simulink model "RefModel_Control"  (R2019b)
settings: Solver=ode1  StartTime=0.0  StopTime=10.0  FixedStep=dt  RelTol=1e-3
(part 2 of 2)

== matlab function RefModel_Control/input_euler_angle_roll_pitch_euler_rate_yaw4 ==
  data: gains_I_pitch data_store_memory; gains_tau_pitch data_store_memory; gains_P_pitch data_store_memory; gains_D_pitch data_store_memory; gains_imax_pitch data_store_memory; gains_FF_pitch data_store_memory; airspeed_min data_store_memory; last_out_pitch data_store_memory; pid_info_I_pitch data_store_memory; pid_info_P_pitch data_store_memory; pid_info_FF_pitch data_store_memory; pid_info_D_pitch data_store_memory; pid_info_desired_pitch data_store_memory; pid_info_actual_pitch data_store_memory; roll data_store_memory; pitch data_store_memory; roll_limit_cd data_store_memory; aspeed data_store_memory; max_rate_neg data_store_memory; gains_rmax_pitch data_store_memory; GRAVITY_MSS data_store_memory; roll_ff_pitch data_store_memory; HD data_store_memory; gains_D_roll data_store_memory; gains_FF_roll data_store_memory; gains_I_roll data_store_memory; gains_imax_roll data_store_memory; gains_P_roll data_store_memory; gains_rmax_roll data_store_memory; gains_tau_roll data_store_memory; last_out_roll data_store_memory; pid_info_actual_roll data_store_memory; pid_info_D_roll data_store_memory; pid_info_desired_roll data_store_memory; pid_info_FF_roll data_store_memory; pid_info_I_roll data_store_memory; pid_info_P_roll data_store_memory; accel_y data_store_memory; imax_yaw data_store_memory; integrator_yaw data_store_memory; K_A_yaw data_store_memory; K_D_last_yaw data_store_memory; K_D_yaw data_store_memory; K_FF_yaw data_store_memory; K_I_yaw data_store_memory; last_out_yaw data_store_memory; last_rate_hp_in_yaw data_store_memory; last_rate_hp_out_yaw data_store_memory; pid_info_D_yaw data_store_memory; pid_info_I_yaw data_store_memory; throttle_dem data_store_memory; pitch_dem data_store_memory; pitch_limit_min_cd data_store_memory; pitch_limit_max_cd data_store_memory; nav_pitch_cd data_store_memory; inverted_flight data_store_memory; k_rudder data_store_memory; k_aileron data_store_memory; k_throttle data_store_memory; k_elevator data_store_memory; kff_throttle_to_pitch data_store_memory; highest_airspeed data_store_memory; scaling_speed data_store_memory; airspeed_max data_store_memory; latAccDem data_store_memory; smoothed_airspeed data_store_memory; aerodynamic_load_factor data_store_memory; kff_rudder_mix data_store_memory; TASmax data_store_memory; SKE_dem data_store_memory; TASmin data_store_memory; SPE_dem data_store_memory; SPE_est data_store_memory; SKE_est data_store_memory; STE_error data_store_memory; SPEdot_dem data_store_memory; SKEdot_dem data_store_memory; STEdot_min data_store_memory; STEdot_max data_store_memory; SPEdot data_store_memory; SKEdot data_store_memory; STEdotErrLast data_store_memory; timeConstant data_store_memory; throttle_cruise data_store_memory; rot_body_to_ned data_store_memory; rollComp data_store_memory; THRmaxf data_store_memory; THRminf data_store_memory; thrDamp data_store_memory; throttle_slewrate data_store_memory; last_throttle_dem data_store_memory; integGain data_store_memory; integTHR_state data_store_memory; maxClimbRate data_store_memory; minSinkRate data_store_memory; EAS_dem data_store_memory; hgt_dem data_store_memory; throttle_max data_store_memory; throttle_min data_store_memory; pitch_max data_store_memory; PITCHmaxf data_store_memory; pitch_min data_store_memory; PITCHminf data_store_memory; pitch_max_limit data_store_memory; TAS_dem data_store_memory; EAS2TAS data_store_memory; TAS_state data_store_memory; integDTAS_state data_store_memory; spdCompFiltOmega data_store_memory; vel_dot data_store_memory; TAS_dem_adj data_store_memory; TAS_rate_dem data_store_memory; hgt_dem_in_old data_store_memory; maxSinkRate data_store_memory; hgt_dem_prev data_store_memory; hgt_dem_adj_last data_store_memory; hgt_dem_adj data_store_memory; hgt_rate_dem data_store_memory; height data_store_memory; climb_rate data_store_memory; spdWeight data_store_memory; ptchDamp data_store_memory; pitch_dem_unc data_store_memory; integSEB_state data_store_memory; vertAccLim data_store_memory; last_pitch_dem data_store_memory; L1_damping data_store_memory; L1_period data_store_memory; current_loc data_store_memory; groundspeed_vector data_store_memory; target_bearing_cd data_store_memory; L1_dist data_store_memory; crosstrack_error data_store_memory; nav_bearing data_store_memory; L1_xtrack_i_gain data_store_memory; L1_xtrack_i_gain_prev data_store_memory; L1_xtrack_i data_store_memory; last_Nu data_store_memory; WPcircle data_store_memory; data_is_stale data_store_memory; bearing_error data_store_memory; LOCATION_SCALING_FACTOR data_store_memory; yaw data_store_memory; reverse data_store_memory; loiter_bank_limit data_store_memory; dt data_store_memory; roll_limit_cd_inint data_store_memory; accel_x data_store_memory; accel_z data_store_memory; Vz data_store_memory; vdot_filter data_store_memory; pwm_min data_store_memory; pwm_max data_store_memory; pwm_out data_store_memory; LOCATION_SCALING_FACTOR_INV data_store_memory; recalc_leash_z data_store_memory; leash_up_z data_store_memory; POSCONTROL_SPEED_UP data_store_memory; POSCONTROL_ACCEL_Z data_store_memory; POSCONTROL_POS_Z_P data_store_memory; leash_down_z data_store_memory; POSCONTROL_SPEED_DOWN data_store_memory; POSCONTROL_ACCELERATION_MIN data_store_memory; POSCONTROL_LEASH_LENGTH_MIN data_store_memory; limit_pos_up data_store_memory; limit_pos_down data_store_memory; pos_error data_store_memory; pos_target data_store_memory; curr_alt data_store_memory; vel_target data_store_memory; limit_vel_up data_store_memory; limit_vel_down data_store_memory; use_desvel_ff_z data_store_memory; reset_rate_to_accel_z data_store_memory; vel_desired data_store_memory; accel_desired data_store_memory; POSCONTROL_VEL_ERROR_CUTOFF_FREQ data_store_memory; vel_last data_store_memory; freeze_ff_z data_store_memory; vel_error data_store_memory; vel_error_input data_store_memory; curr_vel data_store_memory; accel_target data_store_memory; POSCONTROL_VEL_Z_P data_store_memory; reset_accel_to_throttle data_store_memory; accel_error data_store_memory; z_accel_meas data_store_memory; pid_accel_z_reset_filter data_store_memory; POSCONTROL_ACC_Z_FILT_HZ data_store_memory; pid_accel_z_input data_store_memory; pid_accel_z_derivative data_store_memory; POSCONTROL_ACC_Z_P data_store_memory; pid_accel_z_integrator data_store_memory; POSCONTROL_ACC_Z_IMAX data_store_memory; throttle_hover data_store_memory; throttle_lower data_store_memory; throttle_upper data_store_memory; POSCONTROL_ACC_Z_D data_store_memory; POSCONTROL_ACC_Z_I data_store_memory; throttle_thrust_max data_store_memory; althold_lean_angle_max data_store_memory; angle_limit_tc data_store_memory; angle_boost_enabled data_store_memory; angle_boost data_store_memory; throttle_rpy_mix data_store_memory; throttle_avg_max data_store_memory; AC_ATTITUDE_CONTROL_ANGLE_LIMIT_THROTTLE_MAX data_store_memory; POSCONTROL_POS_XY_P data_store_memory; curr_pos data_store_memory; leash data_store_memory; POSCONTROL_ACCEL_XY data_store_memory; POSCONTROL_VEL_XY_FILT_HZ data_store_memory; POSCONTROL_VEL_XY_FILT_D_HZ data_store_memory; pid_vel_xy_reset_filter data_store_memory; pid_vel_xy_input data_store_memory; pid_vel_xy_derivative data_store_memory; pid_vel_xy_integrator data_store_memory; POSCONTROL_VEL_XY_P data_store_memory; limit_accel_xy data_store_memory; motors_limit_throttle_upper data_store_memory; POSCONTROL_VEL_XY_I data_store_memory; POSCONTROL_VEL_XY_IMAX data_store_memory; POSCONTROL_VEL_XY_D data_store_memory; reset_accel_to_lean_xy data_store_memory; POSCONTROL_ACCEL_FILTER_HZ data_store_memory; accel_xy_input data_store_memory; accel_xy_angle_max data_store_memory; roll_target data_store_memory; pitch_target data_store_memory; POSCONTROL_ACCEL_XY_MAX data_store_memory; recalc_leash_xy data_store_memory; POSCONTROL_SPEED data_store_memory; reset_desired_vel_to_pos data_store_memory; POSCONTROL_OVERSPEED_GAIN_Z data_store_memory; POSCONTROL_JERK_RATIO data_store_memory; accel_last_z_cms data_store_memory; is_active_z data_store_memory; POSCONTROL_STOPPING_DIST_DOWN_MAX data_store_memory; POSCONTROL_STOPPING_DIST_UP_MAX data_store_memory; is_active_xy data_store_memory; attitude_target_quat data_store_memory; attitude_target_ang_vel data_store_memory; thrust_error_angle data_store_memory; rate_target_ang_vel data_store_memory; gyro_z data_store_memory; ang_vel_roll_max data_store_memory; ang_vel_pitch_max data_store_memory; ang_vel_yaw_max data_store_memory; AC_ATTITUDE_THRUST_ERROR_ANGLE data_store_memory; rate_bf_ff_enabled data_store_memory; attitude_ang_error data_store_memory; p_angle_yaw data_store_memory; AC_ATTITUDE_ACCEL_Y_CONTROLLER_MAX_RADSS data_store_memory; use_sqrt_controller data_store_memory; p_angle_roll data_store_memory; AC_ATTITUDE_ACCEL_RP_CONTROLLER_MIN_RADSS data_store_memory; AC_ATTITUDE_ACCEL_RP_CONTROLLER_MAX_RADSS data_store_memory; p_angle_pitch data_store_memory; accel_pitch_max data_store_memory; accel_yaw_max data_store_memory; accel_roll_max data_store_memory; AC_ATTITUDE_ACCEL_Y_CONTROLLER_MIN_RADSS data_store_memory; attitude_target_euler_angle data_store_memory; input_tc data_store_memory; attitude_target_euler_rate data_store_memory; slew_yaw data_store_memory; rate_pitch_pid_reset_filter data_store_memory; rate_pitch_pid_input data_store_memory; rate_pitch_pid_derivative data_store_memory; rate_pitch_pid_integrator data_store_memory; motors_limit_roll_pitch data_store_memory; ATC_RAT_PIT_D data_store_memory; ATC_RAT_PIT_FF data_store_memory; ATC_RAT_PIT_FILT data_store_memory; ATC_RAT_PIT_I data_store_memory; ATC_RAT_PIT_IMAX data_store_memory; ATC_RAT_PIT_P data_store_memory; ATC_RAT_RLL_D data_store_memory; ATC_RAT_RLL_FF data_store_memory; ATC_RAT_RLL_FILT data_store_memory; ATC_RAT_RLL_I data_store_memory; ATC_RAT_RLL_IMAX data_store_memory; ATC_RAT_RLL_P data_store_memory; rate_roll_pid_reset_filter data_store_memory; rate_roll_pid_input data_store_memory; rate_roll_pid_derivative data_store_memory; rate_roll_pid_integrator data_store_memory; ATC_RAT_YAW_D data_store_memory; ATC_RAT_YAW_FF data_store_memory; ATC_RAT_YAW_FILT data_store_memory; ATC_RAT_YAW_I data_store_memory; ATC_RAT_YAW_IMAX data_store_memory; ATC_RAT_YAW_P data_store_memory; rate_yaw_pid_reset_filter data_store_memory; rate_yaw_pid_input data_store_memory; rate_yaw_pid_derivative data_store_memory; rate_yaw_pid_integrator data_store_memory; motors_limit_yaw data_store_memory; gyro_x data_store_memory; gyro_y data_store_memory; inint data_store_memory; AP_MOTORS_MATRIX_YAW_FACTOR_CCW data_store_memory; AP_MOTORS_MATRIX_YAW_FACTOR_CW data_store_memory; pitch_factor data_store_memory; roll_factor data_store_memory; yaw_factor data_store_memory; throttle_in data_store_memory; throttle_cutoff_frequency data_store_memory; POSCONTROL_THROTTLE_CUTOFF_FREQ data_store_memory; throttle_filter data_store_memory; armed data_store_memory; roll_in data_store_memory; pitch_in data_store_memory; yaw_in data_store_memory; thrust_boost_ratio data_store_memory; thrust_rpyt_out data_store_memory; limit_roll_pitch data_store_memory; yaw_headroom data_store_memory; thrust_boost data_store_memory; limit_yaw data_store_memory; current_tilt data_store_memory; air_density_ratio data_store_memory; thrust_slew_time data_store_memory; attitude_error_vector data_store_memory; Kx data_store_memory; target_yaw_rate data_store_memory; climb_rate_cms data_store_memory; mode data_store_memory; mode_L1 data_store_memory; hgt_dem_cm data_store_memory; EAS_dem_cm data_store_memory; arspeed_filt data_store_memory; arspeed_temp data_store_memory; loc_origin data_store_memory; roll_target_pilot data_store_memory; pitch_target_pilot data_store_memory; center_WP data_store_memory; radius data_store_memory; loiter_direction data_store_memory; prev_WP data_store_memory; next_WP data_store_memory; dist_min data_store_memory; L1_radius data_store_memory; loc data_store_memory; tail_tilt data_store_memory; p_tail_tilt data_store_memory; p_tilt_pitch_target data_store_memory; disable_integrator_pitch data_store_memory; disable_integrator_roll data_store_memory; disable_integrator_yaw data_store_memory; aspeed_c2p data_store_memory; p_plane_c2p data_store_memory; yaw_max_c2p data_store_memory; weathervane_min_roll data_store_memory; weathervane_gain data_store_memory; yaw_rate_max data_store_memory; weathervane_last_output data_store_memory; POSCONTROL_ACC_Z_FILT_HZ_c2p data_store_memory; nav_roll_cd data_store_memory
function input_euler_angle_roll_pitch_euler_rate_yaw
global aerodynamic_load_factor
global roll_target
global pitch_target
global target_yaw_rate
global throttle_in
global climb_rate_cms
global mode
persistent mode_state
global POSCONTROL_THROTTLE_CUTOFF_FREQ
global inint
global dt
global height
%%%%%%%%%%%%%%%%%%%%%%%%%%%%%%%
global pos_target
global curr_alt
global curr_pos
global loc_origin
global current_loc
global EAS_dem_cm
global hgt_dem_cm
global hgt_dem
global arspeed_filt
global aspeed
global arspeed_temp
global p_tilt_pitch_target
global tail_tilt
%%%%%%%%%%%%%%%%%%%%%%%%%%%%%%%%%%
global roll_target_pilot
global pitch_target_pilot
global vel_desired
global yaw
%%%%%%%%%%L1%%%%%%%%%%%%%%%%%%%%%
global center_WP
global radius
global loiter_direction
global prev_WP
global next_WP
global dist_min
global loc
global L1_radius
persistent WP_i
%%%%%%%%%%%%%%%%%%%%%%%%%%%%%%%
global disable_integrator_pitch
global disable_integrator_roll
global disable_integrator_yaw
global aspeed_c2p
global k_aileron 
global k_elevator 
global k_rudder 
global nav_pitch_cd
global nav_roll_cd
global roll_in
global pitch_in
global yaw_in
global p_plane_c2p
global yaw_max_c2p
global roll_ff_pitch
global K_FF_yaw
global attitude_target_quat
global rot_body_to_ned
persistent POSCONTROL_ACC_Z_FILT_HZ_inint
global POSCONTROL_ACC_Z_FILT_HZ
global POSCONTROL_ACC_Z_FILT_HZ_c2p
%%%%%%%%%%%%%%%%%%%%%%%%%%%%%%%%
  if(mode==5||mode==6||mode==4)
    disable_integrator_pitch=0;
    disable_integrator_roll=0;
    disable_integrator_yaw=0;
    roll_ff_pitch=1;
    K_FF_yaw=1;
  else
    disable_integrator_pitch=1;
    disable_integrator_roll=1;
    disable_integrator_yaw=1;
    roll_ff_pitch=0;
    K_FF_yaw=0;
  end

    if isempty(mode_state)
        mode_state = 0;
    end
    
    if isempty(WP_i)
        WP_i = 1;
    end  
    
    if isempty(POSCONTROL_ACC_Z_FILT_HZ_inint)
        POSCONTROL_ACC_Z_FILT_HZ_inint = POSCONTROL_ACC_Z_FILT_HZ;
    end  
    
    if(inint)
    setup_motors() ;
    inint=0;
    end

  %% mode 1 :copter Stabilize,2:copter althold ,3:copter poshold,4:Plane Stabilize 5:Plane TECS; 6：Plane L1  
  updata_cl();
  rc=1/(2*pi*arspeed_filt);
  alpha=dt/(dt+rc);
  arspeed_temp=arspeed_temp+(aspeed-arspeed_temp)*alpha;
  aspeed=arspeed_temp;
  

switch mode
    case 1 %copter Stabilize
        if(mode_state~=1)
            attitude_target_quat=from_rotation_matrix(rot_body_to_ned);%20200225  
            mode_state=1;
        end                
        set_throttle_out(throttle_in, 1, POSCONTROL_THROTTLE_CUTOFF_FREQ);
        input_euler_angle_roll_pitch_euler_rate_yaw(  roll_target,   pitch_target,   target_yaw_rate);
        rate_controller_run();
        AP_MotorsMulticopter_output();
    case 2 %copter althold
        if(mode_state~=2)
            pos_target(3) = curr_alt;
            mode_state=2;            
        end
         set_alt_target_from_climb_rate_ff(climb_rate_cms, dt, 0)
         update_z_controller();
          input_euler_angle_roll_pitch_euler_rate_yaw(  roll_target,   pitch_target,   target_yaw_rate);
         rate_controller_run();
         AP_MotorsMulticopter_output();
    case 3 %copter xyz
        if(mode_state~=3)
            loc_origin=current_loc;
            curr_pos(1:2)=[0 0];
            pos_target(1:2)=[0 0];
            pos_target(3) = curr_alt;
            mode_state=3;
        else
%             pos_target(1:2)=[0 0];
            curr_pos(1:2)=get_vector_xy_from_origin_NE( current_loc,loc_origin)*100; 
        end
         vel_desired(1)=pitch_target_pilot/10*cos(yaw)-roll_target_pilot/10*sin(yaw);
         vel_desired(2)=pitch_target_pilot/10*sin(yaw)+roll_target_pilot/10*cos(yaw);
         
         if( (abs(pitch_target_pilot)>0) || (abs(roll_target_pilot)>0)||(abs(target_yaw_rate)>0))
             temp_yaw_rate=0;
         else
             temp_yaw_rate=get_weathervane_yaw_rate_cds();
         end                 
         set_alt_target_from_climb_rate_ff(climb_rate_cms, dt, 0)
         update_vel_controller_xy();
         update_z_controller();
         input_euler_angle_roll_pitch_euler_rate_yaw(  roll_target,   pitch_target,   target_yaw_rate+temp_yaw_rate);
         rate_controller_run();
         AP_MotorsMulticopter_output();
    case 4 %Plane Stabilize
        if(mode_state~=4)         
            mode_state=4;
        end
%         calc_nav_pitch();
        calc_nav_roll()
        calc_throttle()
        stabilize()
        output_to_motors_plane();
    case 5 %Plane TECS
        if(mode_state~=5)
            hgt_dem_cm=height*100;
            hgt_dem=height;
            mode_state=5;
        else
            hgt_dem_cm=hgt_dem_cm+dt*climb_rate_cms;
        end    
        update_50hz();
        update_pitch_throttle(  hgt_dem_cm,EAS_dem_cm,aerodynamic_load_factor)
        %update_loiter( center_WP,   radius,   loiter_direction)
        %update_waypoint( prev_WP,  next_WP,  dist_min)
        calc_nav_pitch();
        calc_nav_roll()
        calc_throttle()
        stabilize()
        output_to_motors_plane();
        %%%%%%%%%%%%%%%%%%%%%%%%%%%%%%%%%%%%%%%%%%%%%
    case 6 %Plane L1 
        if(mode_state~=6)
             mode_state=6;  
             hgt_dem_cm=height*100;
             hgt_dem=height;
        else
             hgt_dem_cm=hgt_dem_cm+dt*climb_rate_cms;

        end    
%         prev_WP=loc(WP_i,2:3);
%         next_WP=loc(WP_i+1,2:3); 
         prev_WP=[loc.lat(WP_i) loc.lon(WP_i)];
         next_WP=[loc.lat(WP_i+1) loc.lon(WP_i+1)];
        
        AB = get_distance_NE(next_WP,current_loc);
        AB_length = norm(AB,2);
        if((AB_length<L1_radius))
            if((loc.num(WP_i+2,1)~=99))       
                WP_i=WP_i+1;      
            else               
                WP_i=2;
            end
        end
        update_50hz();
        update_pitch_throttle(  hgt_dem_cm,EAS_dem_cm,aerodynamic_load_factor)
%         update_loiter( center_WP,   radius,   loiter_direction)
         update_waypoint( prev_WP,  next_WP,  dist_min)
        calc_nav_pitch();
        calc_nav_roll()
        calc_throttle()
        stabilize()
        output_to_motors_plane();
    case 7 %copter althold
        if(mode_state~=7)
            pos_target(3) = curr_alt;
            mode_state=7;
         attitude_target_quat=from_rotation_matrix(rot_body_to_ned);%20200225
        end
         set_alt_target_from_climb_rate_ff(climb_rate_cms, dt, 0)
         update_z_controller();
         tail_tilt_temp=constrain_value(tail_tilt,-3000,700);
         pitch_target_temp=pitch_target+p_tilt_pitch_target*tail_tilt_temp;
         input_euler_angle_roll_pitch_euler_rate_yaw(  roll_target,   pitch_target_temp,   target_yaw_rate);
         rate_controller_run();
         if(aspeed>aspeed_c2p)
            nav_pitch_cd=pitch_target;
            nav_roll_cd=roll_target;
            stabilize()
            k_aileron=k_aileron*p_plane_c2p;
            k_elevator=k_elevator*p_plane_c2p;
            k_rudder=k_rudder*p_plane_c2p;
            yaw_in=constrain_value(yaw_in,-yaw_max_c2p,yaw_max_c2p);
            POSCONTROL_ACC_Z_FILT_HZ=POSCONTROL_ACC_Z_FILT_HZ_c2p;
            
         else
             
             POSCONTROL_ACC_Z_FILT_HZ=POSCONTROL_ACC_Z_FILT_HZ_inint;
             k_aileron=0;
             k_elevator=0;
             k_rudder=0;
         end
        AP_MotorsMulticopter_output();
    otherwise  %copter Stabilize
%         set_throttle_out(throttle_in, 1, POSCONTROL_THROTTLE_CUTOFF_FREQ);
%         input_euler_angle_roll_pitch_euler_rate_yaw(  roll_target,   pitch_target,   target_yaw_rate);
%         rate_controller_run();
%         AP_MotorsMulticopter_output();
end
    

%%%%%%%%%%%%%%%%%%%%%%%%%%%%%%%%%%%%%%%%%%%%%%%%%%%%%%%%%%%%%%%%%%%%%%%%%%%%%%%%%
